simulink model "Tester_Blocks"  (R2024b)
settings: Solver=FixedStepAuto  StartTime=0  StopTime=60  FixedStep=0.001  RelTol=1e-3
values from neighbouring files (symbols this model uses):
  motor_B = 0.0001    [Lab1_motor_params_student.m]    (also in Lab1_motor_params_student_multi.m)
  motor_Eff = 0.5    [Lab1_motor_params_student.m]    (also in Lab1_motor_params_student_multi.m)
  motor_J = 0.001    [Lab1_motor_params_student.m]    (also in Lab1_motor_params_student_multi.m)
  motor_Ke = 0.05    [Lab1_motor_params_student.m]    (also in Lab1_motor_params_student_multi.m)
  motor_L = 0.0254006445    [Lab1_motor_params_student.m]    (also in Lab1_motor_params_student_multi.m = 0.0291360334)
  motor_R = 0.98275    [Lab1_motor_params_student.m]    (also in Lab1_motor_params_student_multi.m = 1.12727)
libraries: simulink x7
settings Model: Creator=tanawatp  LastModifiedBy=acer
settings RTWCC: GPUComputeCapability=3.5

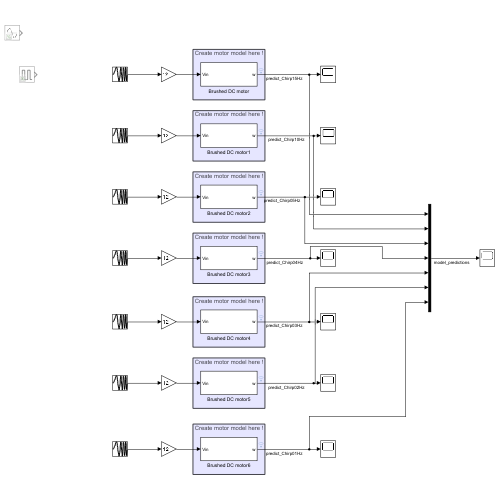
[thumbnail: Simulink's stored preview of the top-level diagram]
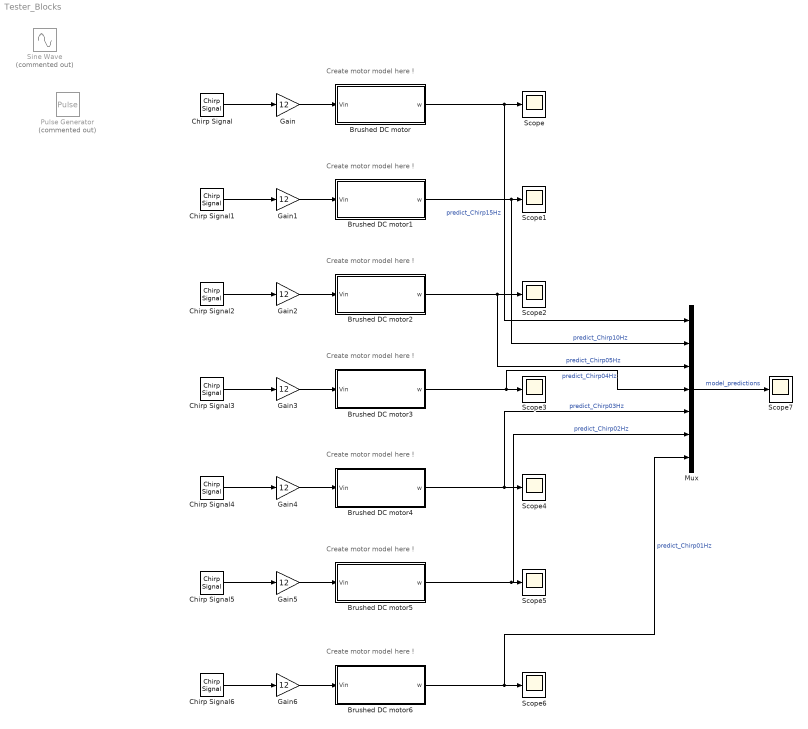
== system Tester_Blocks ==
  note: Create motor model here !
  note: Create motor model here !
  note: Create motor model here !
  note: Create motor model here !
  note: Create motor model here !
  note: Create motor model here !
  note: Create motor model here !
  Brushed DC motor : Subsystem
  Brushed DC motor1 : Subsystem
  Brushed DC motor2 : Subsystem
  Brushed DC motor3 : Subsystem
  Brushed DC motor4 : Subsystem
  Brushed DC motor5 : Subsystem
  Brushed DC motor6 : Subsystem
  Chirp Signal : simulink/Sources/Chirp Signal  f1=0  T=60  f2=1.5
  Chirp Signal1 : simulink/Sources/Chirp Signal  f1=0  T=60  f2=1
  Chirp Signal2 : simulink/Sources/Chirp Signal  f1=0  T=60  f2=0.5
  Chirp Signal3 : simulink/Sources/Chirp Signal  f1=0  T=60  f2=0.4
  Chirp Signal4 : simulink/Sources/Chirp Signal  f1=0  T=60  f2=0.3
  Chirp Signal5 : simulink/Sources/Chirp Signal  f1=0  T=60  f2=0.2
  Chirp Signal6 : simulink/Sources/Chirp Signal  f1=0  T=60  f2=0.1
  Gain{,1..6} (7 alike) : Gain  Gain=12
  Mux : Mux  Inputs=7
  Pulse Generator : DiscretePulseGenerator  Commented=on  PulseType=Time based  PulseWidth=50
  Scope{,1..7} (8 alike) : Scope
  Sine Wave : Sin  Commented=on  Frequency=0.2  SampleTime=0
  wires:
  Brushed DC motor/1(w) -> Mux/1, Scope/1  "predict_Chirp15Hz"
  Chirp Signal/1 -> Gain/1
  Gain/1 -> Brushed DC motor/1(Vin)
  Gain1/1 -> Brushed DC motor1/1(Vin)
  Chirp Signal1/1 -> Gain1/1
  Brushed DC motor1/1(w) -> Mux/2, Scope1/1  "predict_Chirp10Hz"
  Brushed DC motor2/1(w) -> Mux/3, Scope2/1  "predict_Chirp05Hz"
  Chirp Signal2/1 -> Gain2/1
  Gain2/1 -> Brushed DC motor2/1(Vin)
  Gain3/1 -> Brushed DC motor3/1(Vin)
  Chirp Signal3/1 -> Gain3/1
  Brushed DC motor3/1(w) -> Mux/4, Scope3/1  "predict_Chirp04Hz"
  Brushed DC motor4/1(w) -> Mux/5, Scope4/1  "predict_Chirp03Hz"
  Chirp Signal4/1 -> Gain4/1
  Gain4/1 -> Brushed DC motor4/1(Vin)
  Gain5/1 -> Brushed DC motor5/1(Vin)
  Chirp Signal5/1 -> Gain5/1
  Brushed DC motor5/1(w) -> Mux/6, Scope5/1  "predict_Chirp02Hz"
  Brushed DC motor6/1(w) -> Mux/7, Scope6/1  "predict_Chirp01Hz"
  Chirp Signal6/1 -> Gain6/1
  Gain6/1 -> Brushed DC motor6/1(Vin)
  Mux/1 -> Scope7/1  "model_predictions"

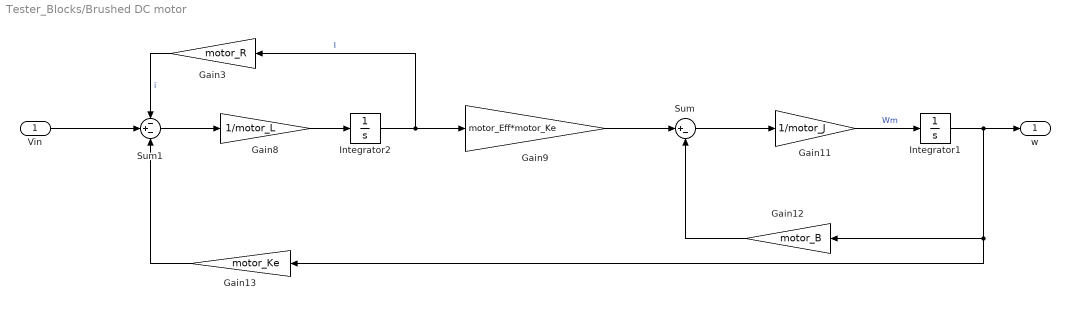
== system Tester_Blocks/Brushed DC motor ==
  Vin : Inport
  Gain11 : Gain  Gain=1/motor_J
  Gain12 : Gain  Gain=motor_B
  Gain13 : Gain  Gain=motor_Ke
  Gain3 : Gain  Gain=motor_R
  Gain8 : Gain  Gain=1/motor_L
  Gain9 : Gain  Gain=motor_Eff*motor_Ke
  Integrator1 : Integrator
  Integrator2 : Integrator
  Sum : Sum  Inputs=|+-
  Sum1 : Sum  Inputs=-+-
  w : Outport
  wires:
  Gain9/1 -> Sum/1
  Sum/1 -> Gain11/1
  Gain12/1 -> Sum/2
  Gain11/1 -> Integrator1/1  "Wm"
  Integrator1/1 -> Gain12/1, Gain13/1, w/1
  Vin/1 -> Sum1/2
  Gain3/1 -> Sum1/1  "i"
  Gain13/1 -> Sum1/3
  Sum1/1 -> Gain8/1
  Gain8/1 -> Integrator2/1
  Integrator2/1 -> Gain3/1, Gain9/1  "I"

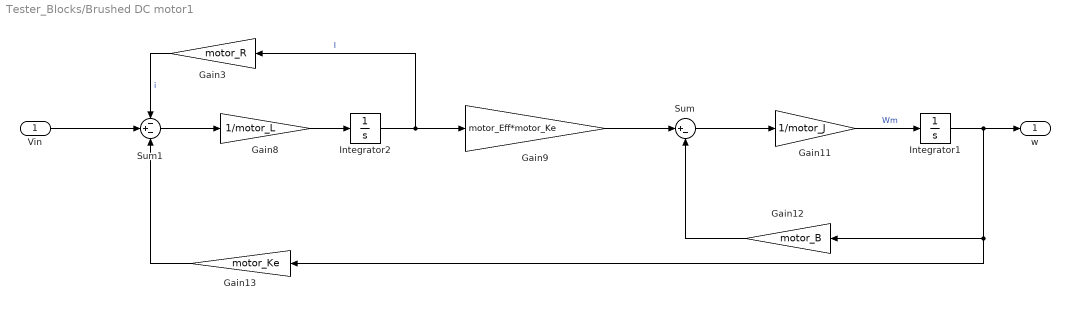
== system Tester_Blocks/Brushed DC motor1 ==
  Vin : Inport
  Gain11 : Gain  Gain=1/motor_J
  Gain12 : Gain  Gain=motor_B
  Gain13 : Gain  Gain=motor_Ke
  Gain3 : Gain  Gain=motor_R
  Gain8 : Gain  Gain=1/motor_L
  Gain9 : Gain  Gain=motor_Eff*motor_Ke
  Integrator1 : Integrator
  Integrator2 : Integrator
  Sum : Sum  Inputs=|+-
  Sum1 : Sum  Inputs=-+-
  w : Outport
  wires:
  Integrator2/1 -> Gain9/1, Gain3/1  "I"
  Gain8/1 -> Integrator2/1
  Sum1/1 -> Gain8/1
  Gain13/1 -> Sum1/3
  Gain3/1 -> Sum1/1  "i"
  Vin/1 -> Sum1/2
  Integrator1/1 -> w/1, Gain13/1, Gain12/1
  Gain11/1 -> Integrator1/1  "Wm"
  Gain12/1 -> Sum/2
  Sum/1 -> Gain11/1
  Gain9/1 -> Sum/1

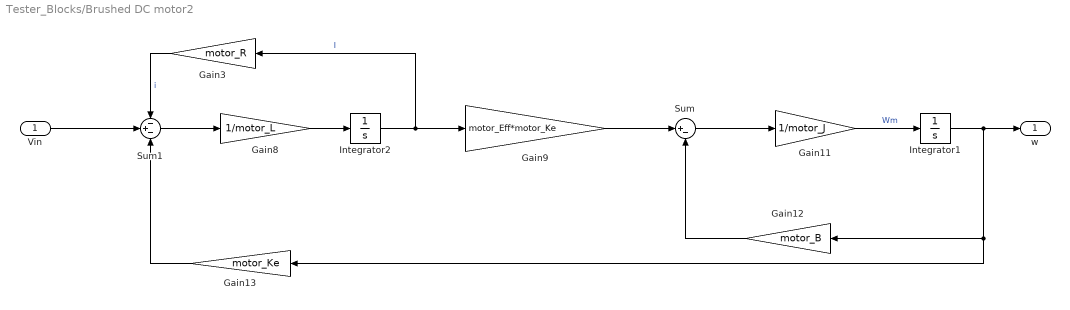
== system Tester_Blocks/Brushed DC motor2 ==
  Vin : Inport
  Gain11 : Gain  Gain=1/motor_J
  Gain12 : Gain  Gain=motor_B
  Gain13 : Gain  Gain=motor_Ke
  Gain3 : Gain  Gain=motor_R
  Gain8 : Gain  Gain=1/motor_L
  Gain9 : Gain  Gain=motor_Eff*motor_Ke
  Integrator1 : Integrator
  Integrator2 : Integrator
  Sum : Sum  Inputs=|+-
  Sum1 : Sum  Inputs=-+-
  w : Outport
  wires:
  Gain9/1 -> Sum/1
  Sum/1 -> Gain11/1
  Gain12/1 -> Sum/2
  Gain11/1 -> Integrator1/1  "Wm"
  Integrator1/1 -> Gain12/1, Gain13/1, w/1
  Vin/1 -> Sum1/2
  Gain3/1 -> Sum1/1  "i"
  Gain13/1 -> Sum1/3
  Sum1/1 -> Gain8/1
  Gain8/1 -> Integrator2/1
  Integrator2/1 -> Gain3/1, Gain9/1  "I"

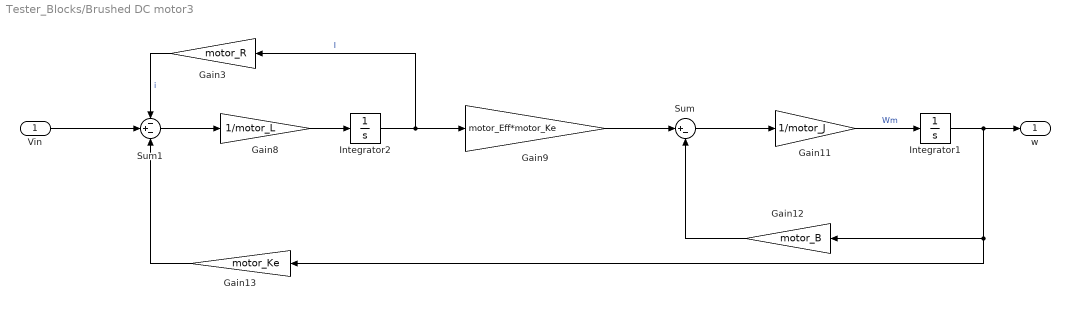
== system Tester_Blocks/Brushed DC motor3 ==
  Vin : Inport
  Gain11 : Gain  Gain=1/motor_J
  Gain12 : Gain  Gain=motor_B
  Gain13 : Gain  Gain=motor_Ke
  Gain3 : Gain  Gain=motor_R
  Gain8 : Gain  Gain=1/motor_L
  Gain9 : Gain  Gain=motor_Eff*motor_Ke
  Integrator1 : Integrator
  Integrator2 : Integrator
  Sum : Sum  Inputs=|+-
  Sum1 : Sum  Inputs=-+-
  w : Outport
  wires:
  Integrator2/1 -> Gain9/1, Gain3/1  "I"
  Gain8/1 -> Integrator2/1
  Sum1/1 -> Gain8/1
  Gain13/1 -> Sum1/3
  Gain3/1 -> Sum1/1  "i"
  Vin/1 -> Sum1/2
  Integrator1/1 -> w/1, Gain13/1, Gain12/1
  Gain11/1 -> Integrator1/1  "Wm"
  Gain12/1 -> Sum/2
  Sum/1 -> Gain11/1
  Gain9/1 -> Sum/1

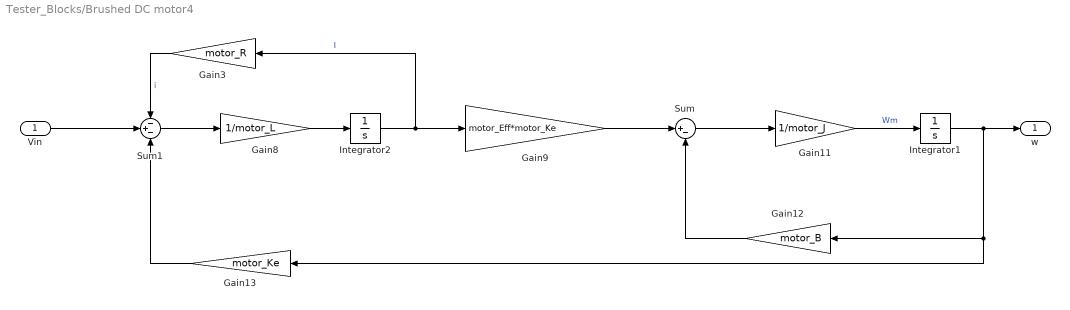
== system Tester_Blocks/Brushed DC motor4 ==
  Vin : Inport
  Gain11 : Gain  Gain=1/motor_J
  Gain12 : Gain  Gain=motor_B
  Gain13 : Gain  Gain=motor_Ke
  Gain3 : Gain  Gain=motor_R
  Gain8 : Gain  Gain=1/motor_L
  Gain9 : Gain  Gain=motor_Eff*motor_Ke
  Integrator1 : Integrator
  Integrator2 : Integrator
  Sum : Sum  Inputs=|+-
  Sum1 : Sum  Inputs=-+-
  w : Outport
  wires:
  Gain9/1 -> Sum/1
  Sum/1 -> Gain11/1
  Gain12/1 -> Sum/2
  Gain11/1 -> Integrator1/1  "Wm"
  Integrator1/1 -> Gain12/1, Gain13/1, w/1
  Vin/1 -> Sum1/2
  Gain3/1 -> Sum1/1  "i"
  Gain13/1 -> Sum1/3
  Sum1/1 -> Gain8/1
  Gain8/1 -> Integrator2/1
  Integrator2/1 -> Gain3/1, Gain9/1  "I"

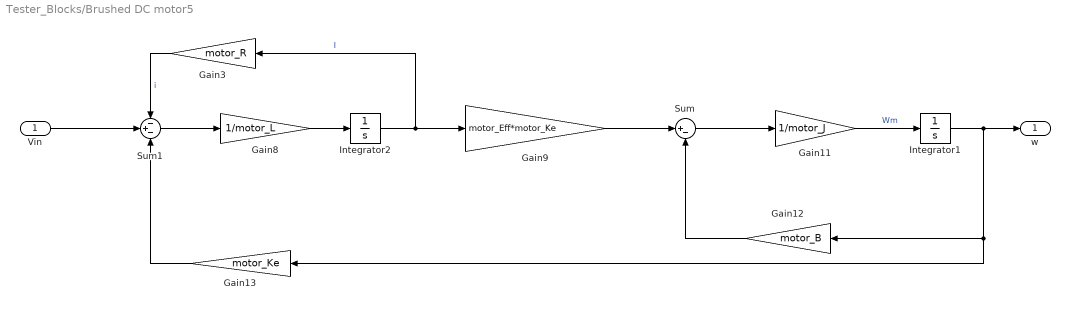
== system Tester_Blocks/Brushed DC motor5 ==
  Vin : Inport
  Gain11 : Gain  Gain=1/motor_J
  Gain12 : Gain  Gain=motor_B
  Gain13 : Gain  Gain=motor_Ke
  Gain3 : Gain  Gain=motor_R
  Gain8 : Gain  Gain=1/motor_L
  Gain9 : Gain  Gain=motor_Eff*motor_Ke
  Integrator1 : Integrator
  Integrator2 : Integrator
  Sum : Sum  Inputs=|+-
  Sum1 : Sum  Inputs=-+-
  w : Outport
  wires:
  Integrator2/1 -> Gain9/1, Gain3/1  "I"
  Gain8/1 -> Integrator2/1
  Sum1/1 -> Gain8/1
  Gain13/1 -> Sum1/3
  Gain3/1 -> Sum1/1  "i"
  Vin/1 -> Sum1/2
  Integrator1/1 -> w/1, Gain13/1, Gain12/1
  Gain11/1 -> Integrator1/1  "Wm"
  Gain12/1 -> Sum/2
  Sum/1 -> Gain11/1
  Gain9/1 -> Sum/1

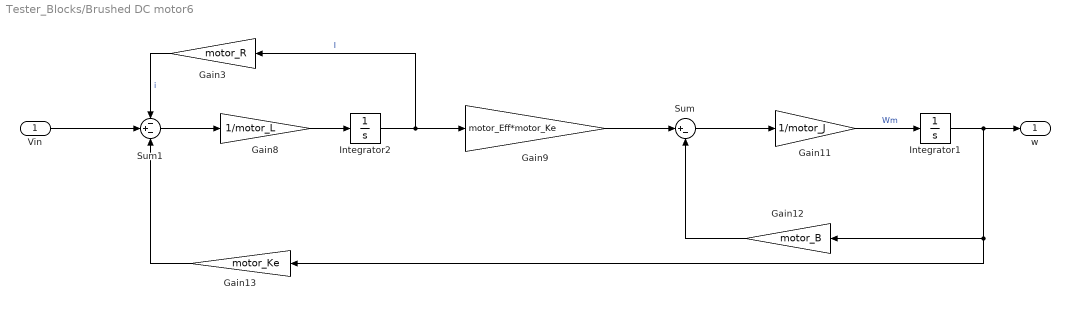
== system Tester_Blocks/Brushed DC motor6 ==
  Vin : Inport
  Gain11 : Gain  Gain=1/motor_J
  Gain12 : Gain  Gain=motor_B
  Gain13 : Gain  Gain=motor_Ke
  Gain3 : Gain  Gain=motor_R
  Gain8 : Gain  Gain=1/motor_L
  Gain9 : Gain  Gain=motor_Eff*motor_Ke
  Integrator1 : Integrator
  Integrator2 : Integrator
  Sum : Sum  Inputs=|+-
  Sum1 : Sum  Inputs=-+-
  w : Outport
  wires:
  Gain9/1 -> Sum/1
  Sum/1 -> Gain11/1
  Gain12/1 -> Sum/2
  Gain11/1 -> Integrator1/1  "Wm"
  Integrator1/1 -> Gain12/1, Gain13/1, w/1
  Vin/1 -> Sum1/2
  Gain3/1 -> Sum1/1  "i"
  Gain13/1 -> Sum1/3
  Sum1/1 -> Gain8/1
  Gain8/1 -> Integrator2/1
  Integrator2/1 -> Gain3/1, Gain9/1  "I"
